simulink model "Hill_muscle_model_simulink"  (R2019a)
settings: Solver=ode45  StartTime=0.0  StopTime=2  FixedStep=0.0001  MaxStep=0.1  RelTol=1e-6  EnableMultiTasking=on
undefined symbols (not defined in the file): prop
(part 3 of 3)

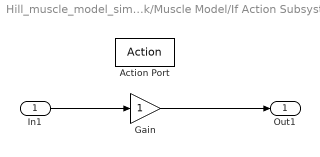
== system Hill_muscle_model_simulink/Muscle Model/If Action Subsystem ==
  In1 : Inport
  Action Port : ActionPort  ActionPortLabel=if(u1 <= +0.02)
  Gain : Gain
  Out1 : Outport
  wires:
  In1/1 -> Gain/1
  Gain/1 -> Out1/1

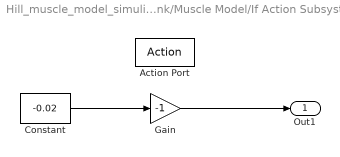
== system Hill_muscle_model_simulink/Muscle Model/If Action Subsystem1 ==
  Action Port : ActionPort  ActionPortLabel=else
  Constant : Constant  Value=-0.02
  Gain : Gain  Gain=-1
  Out1 : Outport  InitialOutput=0.001
  wires:
  Constant/1 -> Gain/1
  Gain/1 -> Out1/1
